simulink model "MPC_Satellite"  (R2021b)
settings: Solver=ode8  StartTime=0.0  StopTime=20  FixedStep=0.001  RelTol=1e-3
InitFcn:
  | GeometricControllerParametersSatellite
values from neighbouring files (symbols this model uses):
  J = diag([22, 20, 23])    [mpc_object.m]
  J_inv = inv(J)    [mpc_object.m]
undefined symbols (not defined in the file or in its folder): FF, g, J2, k_v, k_x, m, mu, normc, Rearth
libraries: robotcorelib x2, mpclib x1
settings Model: Creator=edgar  LastModifiedBy=lapyr
settings SolverCC: ZeroCrossAlgorithm=Adaptive  AlgebraicLoopSolver=LineSearch
settings DebuggingCC: IgnoredZcDiagnostic=none
settings SFSimCC: CustomCodeUndefinedFunction=UseInterfaceOnly
settings RTWCC: DLArmComputeVersion=20.02.1

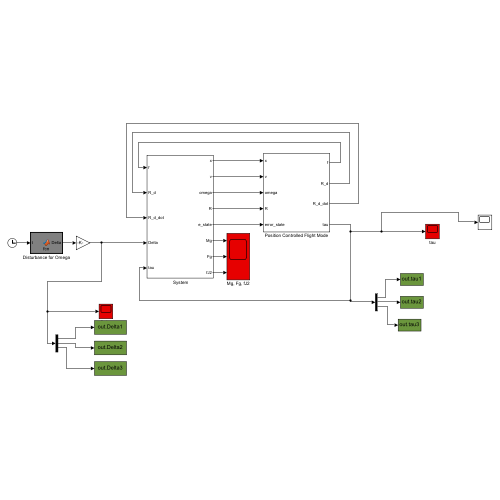
[thumbnail: Simulink's stored preview of the top-level diagram]
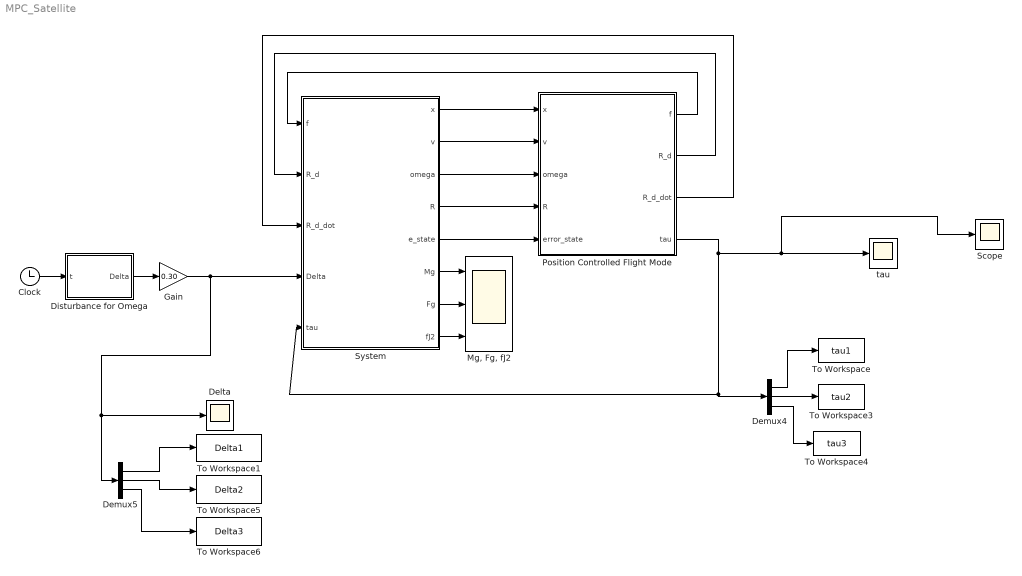
== system MPC_Satellite ==
  " System " : Subsystem
  Clock : Clock
  Delta : Scope
  Demux4 : Demux  Outputs=3
  Demux5 : Demux  Outputs=3
  Disturbance for Omega : MATLAB Function  TreatAsAtomicUnit=on
  Gain : Gain  Gain=0.30
  "Mg, Fg, fJ2" : Scope  NumInputPorts=3
  "Position Controlled Flight Mode " : Subsystem
  Scope : Scope
  To Workspace : ToWorkspace  VariableName=tau1  SaveFormat=Timeseries  SampleTime=-1
  To Workspace1 : ToWorkspace  VariableName=Delta1  SaveFormat=Timeseries  SampleTime=-1
  To Workspace3 : ToWorkspace  VariableName=tau2  SaveFormat=Timeseries  SampleTime=-1
  To Workspace4 : ToWorkspace  VariableName=tau3  SaveFormat=Timeseries  SampleTime=-1
  To Workspace5 : ToWorkspace  VariableName=Delta2  SaveFormat=Timeseries  SampleTime=-1
  To Workspace6 : ToWorkspace  VariableName=Delta3  SaveFormat=Timeseries  SampleTime=-1
  tau : Scope
  wires:
  "Position Controlled Flight Mode "/1(f) -> " System "/1(f)
  Demux4/1 -> To Workspace/1
  Demux4/2 -> To Workspace3/1
  Demux4/3 -> To Workspace4/1
  "Position Controlled Flight Mode "/4(tau) -> Scope/1, tau/1, Demux4/1, " System "/5(tau)
  " System "/4(R) -> "Position Controlled Flight Mode "/4(R)
  "Position Controlled Flight Mode "/2(R_d) -> " System "/2(R_d)
  "Position Controlled Flight Mode "/3(R_d_dot) -> " System "/3(R_d_dot)
  " System "/3(omega) -> "Position Controlled Flight Mode "/3(omega)
  " System "/5(e_state) -> "Position Controlled Flight Mode "/5(error_state)
  " System "/6(Mg) -> "Mg, Fg, fJ2"/1
  " System "/7(Fg) -> "Mg, Fg, fJ2"/2
  " System "/8(fJ2) -> "Mg, Fg, fJ2"/3
  " System "/1(x) -> "Position Controlled Flight Mode "/1(x)
  " System "/2(v) -> "Position Controlled Flight Mode "/2(v)
  Clock/1 -> Disturbance for Omega/1(t)
  Disturbance for Omega/1(Delta) -> Gain/1
  Gain/1 -> Delta/1, Demux5/1, " System "/4(Delta)
  Demux5/3 -> To Workspace6/1
  Demux5/2 -> To Workspace5/1
  Demux5/1 -> To Workspace1/1

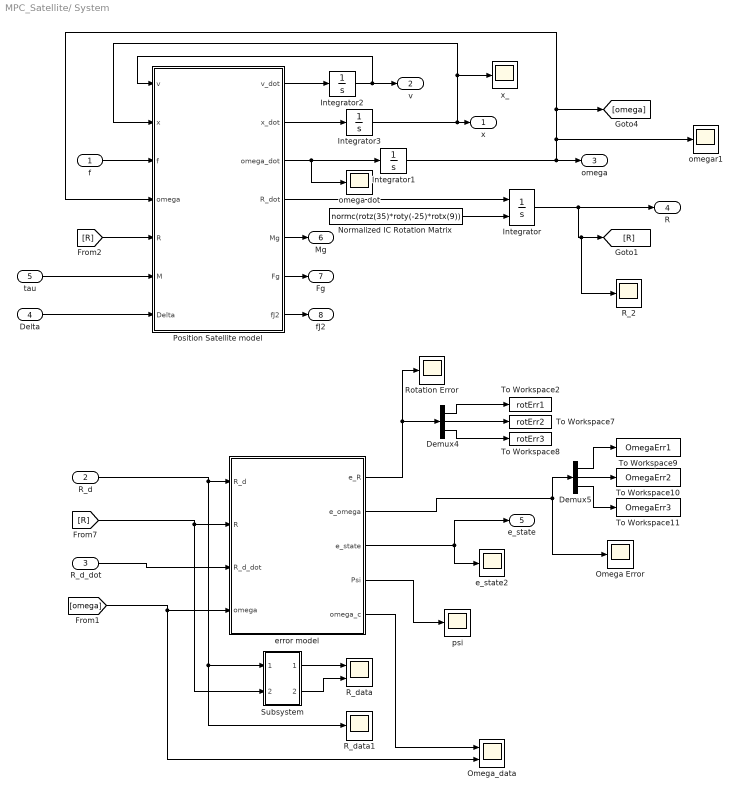
== system MPC_Satellite/ System  ==
  f : Inport
  R_d : Inport  Port=2
  R_d_dot : Inport  Port=3
  Delta : Inport  Port=4
  tau : Inport  Port=5
  Demux4 : Demux  Outputs=3
  Demux5 : Demux  Outputs=3
  Integrator : Integrator  InitialConditionSource=external  InitialCondition=eye(3)
  Integrator1 : Integrator  InitialCondition=[1;1;1]
  Integrator2 : Integrator  InitialCondition=[2;3;4]
  Integrator3 : Integrator  InitialCondition=[90;110;115]
  "Normalized IC Rotation Matrix " : Constant  Value=normc(rotz(35)*roty(-25)*rotx(9))
  Omega Error : Scope
  Omega_data : Scope  NumInputPorts=2
  Position Satellite model : MATLAB Function  TreatAsAtomicUnit=on
  R_2 : Scope
  R_data : Scope  NumInputPorts=2
  R_data1 : Scope
  Rotation Error : Scope
  Subsystem : Subsystem
  To Workspace10 : ToWorkspace  VariableName=OmegaErr2  SaveFormat=Timeseries  SampleTime=-1
  To Workspace11 : ToWorkspace  VariableName=OmegaErr3  SaveFormat=Timeseries  SampleTime=-1
  To Workspace2 : ToWorkspace  VariableName=rotErr1  SaveFormat=Timeseries  SampleTime=-1
  To Workspace7 : ToWorkspace  VariableName=rotErr2  SaveFormat=Timeseries  SampleTime=-1
  To Workspace8 : ToWorkspace  VariableName=rotErr3  SaveFormat=Timeseries  SampleTime=-1
  To Workspace9 : ToWorkspace  VariableName=OmegaErr1  SaveFormat=Timeseries  SampleTime=-1
  e_state2 : Scope
  error model : MATLAB Function  TreatAsAtomicUnit=on
  omega dot : Scope
  omegar1 : Scope
  psi : Scope
  x_ : Scope
  x : Outport
  v : Outport  Port=2
  omega : Outport  Port=3
  R : Outport  Port=4
  e_state : Outport  Port=5
  Mg : Outport  Port=6
  Fg : Outport  Port=7
  fJ2 : Outport  Port=8
  wires:
  Integrator3/1 -> x_/1, Position Satellite model/2(x), x/1
  Position Satellite model/1(v_dot) -> Integrator2/1
  Integrator/1 -> R_2/1, [R], R/1
  Position Satellite model/4(R_dot) -> Integrator/1
  Integrator1/1 -> [omega], Position Satellite model/4(omega), omegar1/1, omega/1
  Integrator2/1 -> Position Satellite model/1(v), v/1
  f/1 -> Position Satellite model/3(f)
  tau/1 -> Position Satellite model/6(M)
  "Normalized IC Rotation Matrix "/1 -> Integrator/2
  Position Satellite model/2(x_dot) -> Integrator3/1
  Demux5/3 -> To Workspace11/1
  Demux5/1 -> To Workspace9/1
  Demux5/2 -> To Workspace10/1
  Demux4/1 -> To Workspace2/1
  Demux4/3 -> To Workspace8/1
  Demux4/2 -> To Workspace7/1
  Position Satellite model/3(omega_dot) -> omega dot/1, Integrator1/1
  [R] -> Subsystem/2(R_d), error model/2(R)
  [omega] -> Omega_data/2, error model/4(omega)
  R_d/1 -> R_data1/1, Subsystem/1(In1), error model/1(R_d)
  R_d_dot/1 -> error model/3(R_d_dot)
  [R] -> Position Satellite model/5(R)
  Position Satellite model/7(fJ2) -> fJ2/1
  Position Satellite model/6(Fg) -> Fg/1
  Position Satellite model/5(Mg) -> Mg/1
  error model/3(e_state) -> e_state/1, e_state2/1
  error model/4(Psi) -> psi/1
  error model/1(e_R) -> Rotation Error/1, Demux4/1
  error model/2(e_omega) -> Omega Error/1, Demux5/1
  Delta/1 -> Position Satellite model/7(Delta)
  Subsystem/1(Out1) -> R_data/1
  Subsystem/2(Out2) -> R_data/2
  error model/5(omega_c) -> Omega_data/1

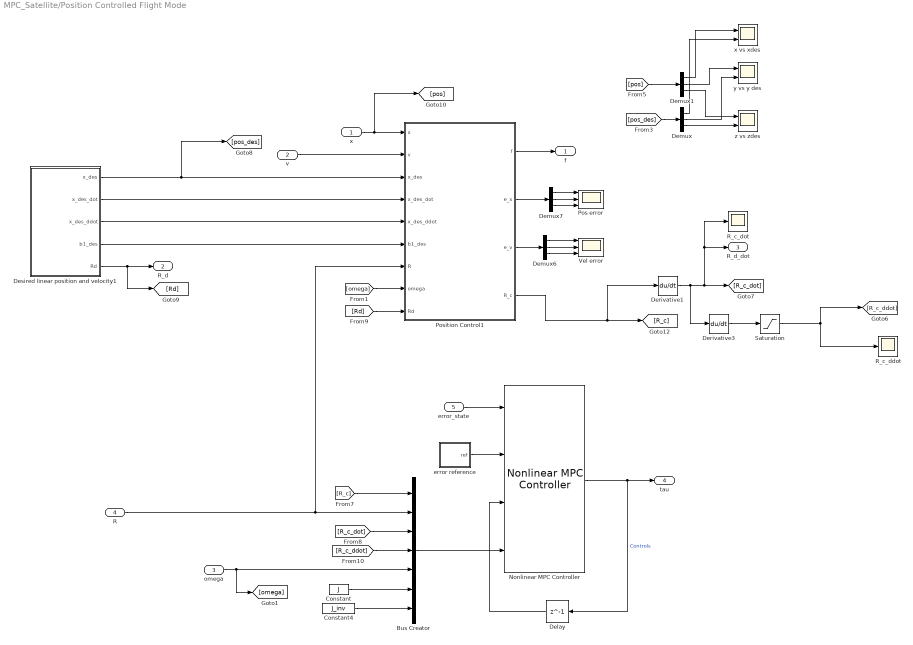
== system MPC_Satellite/Position Controlled Flight Mode  ==
  x : Inport
  v : Inport  Port=2
  omega : Inport  Port=3
  R : Inport  Port=4
  error_state : Inport  Port=5
  Bus Creator : BusCreator  Inputs=7  OutDataTypeStr=Bus: myBusObject  NonVirtualBus=on
      settings: InheritFromInputs=off
  Constant : Constant  Value=J
  Constant4 : Constant  Value=J_inv
  Delay : Delay  DelayLength=1  InitialCondition=0
  Demux{,1,6..7} (4 alike) : Demux  Outputs=3
  Derivative1 : Derivative
  Derivative3 : Derivative
  Desired linear position and velocity1 : Subsystem
  Nonlinear MPC Controller : mpclib/Nonlinear MPC Controller  SCDEnableBlockLinearizationSpecification=on  nlmpcobj=nlobj  UseObjectTs=on  UseMEX=off  md_enabled=off  mvtarget_enabled=off  param_enabled=on  cost_enabled=off  mvseq_enabled=off  stateseq_enabled=off  ovseq_enabled=off  slack_enabled=off  status_enabled=off  ov_min=off  ov_max=off  mv_min=off  mv_max=off  mvrate_min=off  mvrate_max=off  state_min=off  state_max=off  ov_weight=off  mv_weight=off  mvrate_weight=off  ecr_weight=off  nlp_initialize=off
  Pos error : Scope  NumInputPorts=3
  Position Control1 : MATLAB Function  TreatAsAtomicUnit=on
  R_c_ddot : Scope
  R_c_dot : Scope
  Saturation : Saturate  UpperLimit=30  LowerLimit=-30
  Vel error : Scope  NumInputPorts=3
  error reference : MATLAB Function  TreatAsAtomicUnit=on
  x vs xdes : Scope  NumInputPorts=2
  y vs y des : Scope  NumInputPorts=2
  z vs zdes : Scope  NumInputPorts=2
  f : Outport
  R_d : Outport  Port=2
  R_d_dot : Outport  Port=3
  tau : Outport  Port=4
  wires:
  [pos_des] -> Demux/1
  [pos] -> Demux1/1
  Demux1/1 -> x vs xdes/1
  Demux/1 -> x vs xdes/2
  Demux1/2 -> y vs y des/1
  Demux/2 -> y vs y des/2
  Demux1/3 -> z vs zdes/1
  Demux/3 -> z vs zdes/2
  error_state/1 -> Nonlinear MPC Controller/1
  Bus Creator/1 -> Nonlinear MPC Controller/4
  error reference/1(ref) -> Nonlinear MPC Controller/2
  Nonlinear MPC Controller/1 -> Delay/1, tau/1  "Controls"
  Delay/1 -> Nonlinear MPC Controller/3
  Constant4/1 -> Bus Creator/7
  [R_c] -> Bus Creator/1
  [R_c_dot] -> Bus Creator/3
  R/1 -> Position Control1/7(R), Bus Creator/2
  [R_c_ddot] -> Bus Creator/4
  omega/1 -> [omega], Bus Creator/5
  Constant/1 -> Bus Creator/6
  [Rd] -> Position Control1/9(Rd)
  [omega] -> Position Control1/8(omega)
  Desired linear position and velocity1/5(Rd) -> [Rd], R_d/1
  Desired linear position and velocity1/3(x_des_ddot) -> Position Control1/5(x_des_ddot)
  Saturation/1 -> R_c_ddot/1, [R_c_ddot]
  Derivative3/1 -> Saturation/1
  Derivative1/1 -> Derivative3/1, R_d_dot/1, R_c_dot/1, [R_c_dot]
  Desired linear position and velocity1/4(b1_des) -> Position Control1/6(b1_des)
  Desired linear position and velocity1/1(x_des) -> [pos_des], Position Control1/3(x_des)
  Position Control1/4(R_c) -> Derivative1/1, [R_c]
  x/1 -> [pos], Position Control1/1(x)
  Position Control1/1(f) -> f/1
  Demux6/2 -> Vel error/2
  Demux6/1 -> Vel error/1
  Demux7/2 -> Pos error/2
  Demux7/3 -> Pos error/3
  Position Control1/3(e_v) -> Demux6/1
  Demux6/3 -> Vel error/3
  Demux7/1 -> Pos error/1
  Position Control1/2(e_x) -> Demux7/1
  Desired linear position and velocity1/2(x_des_dot) -> Position Control1/4(x_des_dot)
  v/1 -> Position Control1/2(v)

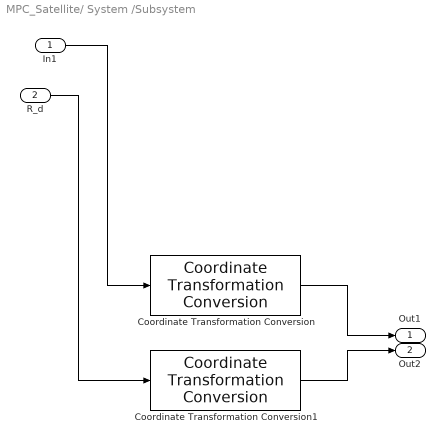
== system MPC_Satellite/ System /Subsystem ==
  In1 : Inport
  R_d : Inport  Port=2
  Coordinate Transformation Conversion : robotcorelib/Coordinate Transformation Conversion  InputRepresentation=Rotation Matrix  InputEulerSequence=ZYX  ShowTrVecInputPort=on  OutputRepresentation=Euler Angles  OutputEulerSequence=XYZ  ShowTrVecOutputPort=on  SimulateUsing=Interpreted execution
      settings: SourceProductBaseCode=NV,RO,RR,UV
  Coordinate Transformation Conversion1 : robotcorelib/Coordinate Transformation Conversion  InputRepresentation=Rotation Matrix  InputEulerSequence=ZYX  ShowTrVecInputPort=on  OutputRepresentation=Euler Angles  OutputEulerSequence=XYZ  ShowTrVecOutputPort=on  SimulateUsing=Interpreted execution
      settings: SourceProductBaseCode=NV,RO,RR,UV
  Out1 : Outport
  Out2 : Outport  Port=2
  wires:
  Coordinate Transformation Conversion1/1 -> Out2/1
  In1/1 -> Coordinate Transformation Conversion/1
  R_d/1 -> Coordinate Transformation Conversion1/1
  Coordinate Transformation Conversion/1 -> Out1/1

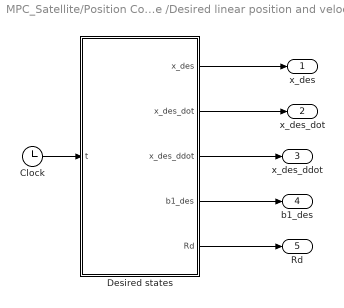
== system MPC_Satellite/Position Controlled Flight Mode /Desired linear position and velocity1 ==
  Clock : Clock
  Desired states : MATLAB Function  TreatAsAtomicUnit=on
  x_des : Outport
  x_des_dot : Outport  Port=2
  x_des_ddot : Outport  Port=3
  b1_des : Outport  Port=4
  Rd : Outport  Port=5
  wires:
  Desired states/1(x_des) -> x_des/1
  Clock/1 -> Desired states/1(t)
  Desired states/2(x_des_dot) -> x_des_dot/1
  Desired states/3(x_des_ddot) -> x_des_ddot/1
  Desired states/5(Rd) -> Rd/1
  Desired states/4(b1_des) -> b1_des/1

== matlab function MPC_Satellite/ System /error model ==
  data: e_R output; e_omega output; e_state output; R_d input; R input; R_d_dot input; omega input; Psi output; omega_c output
function [ e_R, e_omega, e_state, Psi,omega_c] = fcn(R_d, R, R_d_dot,omega)

    omega_c_hat =  R_d' * R_d_dot ;           %(22)
    omega_c = [omega_c_hat(3,2); - omega_c_hat(3,1); omega_c_hat(2,1)];
            
    R_mul = (R_d'*R) - (R'*R_d);
    R_mul_vect = [R_mul(3,2); -R_mul(3,1); R_mul(2,1)];
    e_R = 0.5 * R_mul_vect;   %(21)   
    e_omega = omega - (R'*R_d*omega_c);  %(21)
    
    
    Psi = (1/2)*trace(eye(3) - R_d'*R);

    e_state = [Psi;e_R;e_omega];

end

== matlab function MPC_Satellite/Position Controlled Flight Mode /Desired linear position and velocity1/Desired states ==
  data: t input; x_des output; x_des_dot output; x_des_ddot output; b1_des output; Rd output
function [x_des, x_des_dot, x_des_ddot, b1_des, Rd] = fcn(t)

% Generar unas trayectorias habituales que deba seguir un satellite
x_des     = [             100 + 0.4*t ; % 4
                          100 + 5*sin(0.7*t) ; % 0.4
                          100 + 0.3*t]; % 0.6

x_des_dot = [               0.4 ; % 4
                            0.7*5*cos(0.7*t); % 0.4*pi = 1.256
                            0.3];% 0.6*pi = 1.88


x_des_ddot = [                0 ; 
                              -0.7^2*5*sin(0.7*t) ; 
                              0];


% Desired orientation for first column of R [ESTE NO SE USA, se deja para otros diseños de control]
b1_des = [  cos(pi*t) ;  
            sin(pi*t) ;
                   0] ;


% Desired orientation
% Modified Rodrigues parameters [MRP] taken from "Predetermined time attitude
% tracking control for rigid spacecraft" in Acta Astronautica'22

sigma_d = 0.01*[cos(0.2*t); 
                sin(0.2*t);
                sin(0.1*t)];

% Transformation from MRP to Quadetrnions:

q0d = (1 - norm(sigma_d)^2)/(1 + norm(sigma_d)^2);
q1d = ( 2*sigma_d(1,1) )/(1 + norm(sigma_d)^2);
q2d = ( 2*sigma_d(2,1) )/(1 + norm(sigma_d)^2);
q3d = ( 2*sigma_d(3,1) )/(1 + norm(sigma_d)^2);

quat_d = [ q0d ,  q1d , q2d , q3d ]';  
quat_d_Normalized = normalize(quat_d);
Rd = quat2rotm(quat_d_Normalized');

== matlab function MPC_Satellite/Position Controlled Flight Mode /error reference ==
  data: ref output
function ref = fcn()

    ref    = zeros(1,7);

end

== matlab function MPC_Satellite/Position Controlled Flight Mode /Position Control1 ==
  data: f output; e_x output; e_v output; R_c output; x input; v input size=[3 1]; x_des input size=[3 1]; x_des_dot input; x_des_ddot input; b1_des input; R input size=[3 3]; omega input; Rd input; k_v parameter; m parameter; e3 parameter; k_x parameter; mu parameter; FF parameter; Rearth parameter; J2 parameter; J parameter
function [f, e_x, e_v, R_c] = fcn( x, v, x_des, x_des_dot, x_des_ddot, b1_des, R, omega, Rd, k_v, m, e3, k_x, mu, FF, Rearth, J2,J)

e_x = x - x_des;   %(17)
e_v = v - R'*x_des_dot;   %(18) x_dot = R*v 

R_B = R'*x;
Fg = - m*(mu/norm(x)^3)*R_B;
fJ2 = - ( (3*m*mu*J2*Rearth^2*R')/(2*norm(x)^5) ) * ( FF - (( 5*(x(3,1))^2 )/( norm(x)^2 ))*eye(3) ) * x  ;

f = - k_x*e_x - k_v*e_v - m*cross(omega, v) + m*x_des_ddot - Fg - fJ2;

% Este lo quito porque es cuando solo tenemos thrust hacia z, asumimos que
% existen controles para el satelite en pares y fuerzas
% aa  = norm( - f );
% b3_c =   -( - f ) / aa ;     %(23)
% 
% a1 = cross( b3_c, b1_des );
% a3 = norm( a1 );
% 
% b1_c = - ( cross(b3_c, a1) ) / a3; %(38)
% 
% a4 = cross(b3_c, b1_c);
% R_c = [b1_c  a4  b3_c];  % (22)

% R_c = eye(3);
R_c = Rd;

== matlab function MPC_Satellite/Disturbance for Omega ==
  data: t input; Delta output
function Delta = fcn(t)

%parameters
kapa1 = 1.2;
kapa2 = 1.1;
kapa3 = 1.3;

%distirbance
Delta = [ kapa1*sin(t); 
          kapa2*cos(t);
          kapa3];

== matlab function MPC_Satellite/ System /Position Satellite model ==
  data: v input size=[3 1]; x input; v_dot output size=[3 1]; f input; x_dot output size=[3 1]; omega_dot output; m parameter; g parameter; omega input; R input; M input; R_dot output; J parameter; J_inv parameter; mu parameter; FF parameter; Rearth parameter; J2 parameter; Mg output; Fg output; fJ2 output; Delta input
function [ v_dot,x_dot,omega_dot,R_dot, Mg,Fg,fJ2] = fcn(v, x, f, m, g,omega,R,M,J, J_inv,mu, FF, Rearth, J2, Delta)

omega_hat = [   0    , -omega(3),  omega(2);
             omega(3),    0     , -omega(1);
            -omega(2), omega(1) ,      0     ];

% Utility terms:
R_B = R'*x;
Mg  = 3*(mu/norm(x)^5)*( cross(R_B, J*R_B) );
Fg  = - m*(mu/norm(x)^3)*R_B;
fJ2 = - ( (3*m*mu*J2*Rearth^2*R')/(2*norm(x)^5) ) * ( FF - (( 5*(x(3,1))^2 )/( norm(x)^2 ))*eye(3) ) * x  ;

% Position
x_dot = R*v;                         
mvDot =  m*cross(omega, v) + Fg + fJ2 + f;                 
v_dot = mvDot/m ;

% Attitude
R_dot = R * omega_hat; 
JomDot = M - cross(omega, J*omega) + Mg  + Delta;
omega_dot = J_inv * JomDot;

%
% omega_dot = J_inv * (M - cross(omega, J*omega)  ) + J_inv * Delta; 
%J_inv es grande, asi que la pert es mas grande de lo que se cree
